simulink model "model_FS_PSH_IEEE39"  (R2020b)
settings: Solver=ode3  StartTime=0.0  StopTime=300  FixedStep=Ts  RelTol=1e-3
PostLoadFcn:
  | IEEE39BusLineLength;
  | vNomHV = 345E3;fNom=60;load('Dynamicload.mat');
InitFcn:
  | IEEE39BusLineLength;
  | vNomHV = 345E3;fNom=60;load('Dynamicload.mat');
values from neighbouring files (symbols this model uses):
  Rp = 0.05    [IEEE39BusLineLength.m]
  t_sw_off = 220    [MAIN_FS_PSH_IEEE39.m]    (also in MAIN_T_PSH_IEEE39.m; MAIN_VS_PSH.m = 45)
  t_sw_on = 130    [MAIN_FS_PSH_IEEE39.m]    (also in MAIN_T_PSH_IEEE39.m; MAIN_VS_PSH.m = 35)
  TL_10_11_len = 14    [IEEE39BusLineLength.m]
  TL_10_13_len = 14    [IEEE39BusLineLength.m]
  TL_13_14_len = 32    [IEEE39BusLineLength.m]
  TL_14_15_len = 70    [IEEE39BusLineLength.m]
  TL_15_16_len = 31.5    [IEEE39BusLineLength.m]
  TL_16_17_len = 26    [IEEE39BusLineLength.m]
  TL_16_19_len = 61    [IEEE39BusLineLength.m]
  TL_16_21_len = 46    [IEEE39BusLineLength.m]
  TL_16_24_len = 15    [IEEE39BusLineLength.m]
  TL_17_18_len = 26    [IEEE39BusLineLength.m]
  TL_17_27_len = 59    [IEEE39BusLineLength.m]
  TL_1_2_len = 134    [IEEE39BusLineLength.m]
  TL_1_39_len = 105    [IEEE39BusLineLength.m]
  TL_21_22_len = 47    [IEEE39BusLineLength.m]
  TL_22_23_len = 33    [IEEE39BusLineLength.m]
  TL_24_23_len = 88    [IEEE39BusLineLength.m]
  TL_25_26_len = 101    [IEEE39BusLineLength.m]
  TL_26_27_len = 46.5    [IEEE39BusLineLength.m]
  TL_26_28_len = 151    [IEEE39BusLineLength.m]
  TL_26_29_len = 200    [IEEE39BusLineLength.m]
  TL_28_29_len = 48    [IEEE39BusLineLength.m]
  TL_2_25_len = 28    [IEEE39BusLineLength.m]
  TL_2_2_len = 49    [IEEE39BusLineLength.m]
  TL_3_18_len = 42    [IEEE39BusLineLength.m]
  TL_3_4_len = 53    [IEEE39BusLineLength.m]
  TL_4_14_len = 33    [IEEE39BusLineLength.m]
  TL_4_5_len = 32.5    [IEEE39BusLineLength.m]
  TL_5_6_len = 14    [IEEE39BusLineLength.m]
  TL_5_8_len = 32    [IEEE39BusLineLength.m]
  TL_6_11_len = 26.5    [IEEE39BusLineLength.m]
  TL_6_7_len = 25.5    [IEEE39BusLineLength.m]
  TL_7_8_len = 15    [IEEE39BusLineLength.m]
  TL_8_9_len = 93    [IEEE39BusLineLength.m]
  TL_9_39_len = 136    [IEEE39BusLineLength.m]
  Ts = 25e-6    (= 2.5e-05)    [MAIN_FS_PSH_IEEE39.m]    (also in MAIN_T_PSH_IEEE39.m; MAIN_VS_PSH.m = 1e-07)
undefined symbols (not defined in the file or in its folder): D1, Delta, FS_PSH, load15, load16, load18, load20, load21, load23, load24, load25, load26, load27, load28, load29, load3, load39, load4, load7, load8
libraries: powerlib x216, sps_avr x10, powerlib_meascontrol x5, pid_lib x1
(part 4 of 8)

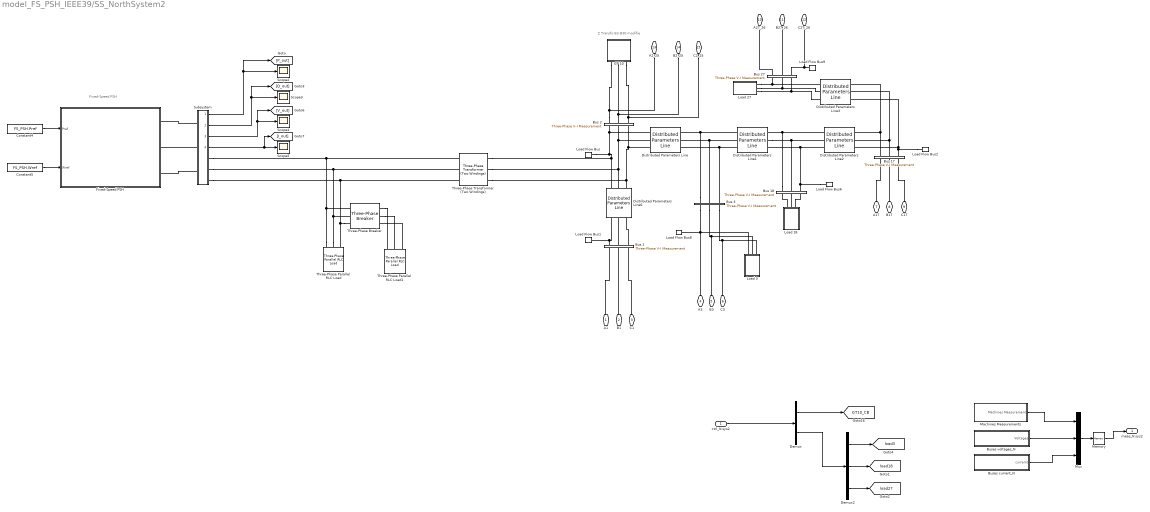
== system model_FS_PSH_IEEE39/SS_NorthSystem2 ==
  note: Z Transfo B2-B30 modifie
  note: Fixed-Speed PSH
  ctrl_N sys2 : Inport
  Bus 1 : powerlib/Measurements/Three-Phase V-I Measurement  VoltageMeasurement=phase-to-ground  SetLabelV=on  LabelV=V_bus_1  Vpu=off  VpuLL=off  CurrentMeasurement=yes  SetLabelI=on  LabelI=I_bus_1  Ipu=off  Pbase=100e6  Vbase=230e3  OutputType=Complex  PhasorSimulation=off  PSBequivalent=0
  Bus 17 : powerlib/Measurements/Three-Phase V-I Measurement  VoltageMeasurement=phase-to-ground  SetLabelV=on  LabelV=V_bus_17  Vpu=off  VpuLL=off  CurrentMeasurement=yes  SetLabelI=on  LabelI=I_bus_17  Ipu=off  Pbase=100e6  Vbase=230e3  OutputType=Complex  PhasorSimulation=off  PSBequivalent=0
  Bus 18 : powerlib/Measurements/Three-Phase V-I Measurement  VoltageMeasurement=phase-to-ground  SetLabelV=on  LabelV=V_bus_18  Vpu=off  VpuLL=off  CurrentMeasurement=yes  SetLabelI=on  LabelI=I_bus_18  Ipu=off  Pbase=100e6  Vbase=230e3  OutputType=Complex  PhasorSimulation=off  PSBequivalent=0
  Bus 2 : powerlib/Measurements/Three-Phase V-I Measurement  VoltageMeasurement=phase-to-ground  SetLabelV=on  LabelV=V_bus_2  Vpu=off  VpuLL=off  CurrentMeasurement=yes  SetLabelI=on  LabelI=I_bus_2  Ipu=off  Pbase=100e6  Vbase=230e3  OutputType=Complex  PhasorSimulation=off  PSBequivalent=0
  Bus 27 : powerlib/Measurements/Three-Phase V-I Measurement  VoltageMeasurement=phase-to-ground  SetLabelV=on  LabelV=V_bus_27  Vpu=off  VpuLL=off  CurrentMeasurement=yes  SetLabelI=on  LabelI=I_bus_27  Ipu=off  Pbase=100e6  Vbase=230e3  OutputType=Complex  PhasorSimulation=off  PSBequivalent=0
  Bus 3 : powerlib/Measurements/Three-Phase V-I Measurement  VoltageMeasurement=phase-to-ground  SetLabelV=on  LabelV=V_bus_3  Vpu=off  VpuLL=off  CurrentMeasurement=yes  SetLabelI=on  LabelI=I_bus_3  Ipu=off  Pbase=100e6  Vbase=230e3  OutputType=Complex  PhasorSimulation=off  PSBequivalent=0
  Buses current_N : Subsystem
  Buses voltages_N : Subsystem
  Constant4 : Constant  Value=FS_PSH.Pref
  Constant5 : Constant  Value=FS_PSH.Wref
  Demux : Demux  Outputs=[1 6]
  Demux2 : Demux  Outputs=[2 2 2]
  Distributed Parameters Line : powerlib/Elements/Distributed Parameters Line  Phases=3  Length=TL_2_2_len  Frequency=fNom  Resistance=[1.547 6.189]/TL_2_2_len  Inductance="[0.048  0.143]/TL_2_2_len"  Capacitance=[0.573e-6 0.261e-6]/TL_2_2_len  x1=[-0.0002 -1.51494241435871e-08 0 0;-0.000175 -1.51813366174431e-08 204759.764947038 -188224.30962879;-0.00015 -1.52119005972007e-08 206524.605301447 -186286.162393846;-0.000125 -1.52411133679905e-08 208271.100946267 -184331.468144834;-0.0001 -1.52689723349653e-08 209999.096747657 -182360.400508997;-7.5e-05 -1.52954750235306e-08 211708.439215037 -180373.134567961;-5e-05 -1.53206190795644e-08 213398.976514727 -178369.846842178;-2.5e-05 -1.53444022696261e-08 215070.558483429 -176350.715275245]  x2=[-0.0002 7.17563772164822e-10 0 0;-0.000175 6.09800920547567e-10 182393.138299879 -200537.913661572;-0.00015 5.0198390288662e-10 184275.023772651 -198810.016888842;-0.000125 3.94122296112896e-10 186140.540872315 -197064.460660873;-0.0001 2.86225681117977e-10 187989.523892855 -195301.400028062;-7.5e-05 1.78303641903076e-10 189821.808596909 -193520.991595647;-5e-05 7.03657647277308e-11 191637.232230355 -191723.393509802;-2.5e-05 -3.75783627416992e-11 193435.633536768 -189908.765443581]  x3=[-0.0002 1.59600858713236e-10 0 0;-0.000175 1.6212940524219e-10 -94.4406795368501 497.211528971884;-0.00015 1.64643550499921e-10 -99.1225635679205 496.299405662674;-0.000125 1.67143071165511e-10 -103.795642959758 495.3431981706;-0.0001 1.69627745217082e-10 -108.459502622431 494.342991431541;-7.5e-05 1.72097351951519e-10 -113.113728284958 493.298874289642;-5e-05 1.74551672004071e-10 -117.757906532103 492.210939489424;-2.5e-05 1.7699048736784e-10 -122.391624841103 491.079283667549]  x4=[-0.0002 -1.7528128884237e-10 0 0;-0.000175 -1.77995252123788e-10 1384.83776478724 -1876.75500949724;-0.00015 -1.80693404837725e-10 1402.46395776973 -1863.6200869169;-0.000125 -1.83375507318658e-10 1419.9655757943 -1850.31962682479;-0.0001 -1.86041321326734e-10 1437.34106426604 -1836.8548106447;-7.5e-05 -1.88690610068941e-10 1454.5888797936 -1823.22683439944;-5e-05 -1.91323138220134e-10 1471.70749032629 -1809.43690860468;-2.5e-05 -1.9393867194394e-10 1488.69537529012 -1795.48625816134]  x5=0.000193191614724863  V1=ones(3,3)  V2=ones(3,3)  I1=ones(3,3)  I2=ones(3,3)  nHarmo=1  Measurements=None  Decoupling=off  VsMag0=0  VrMag0=0  VsAngle0=0  VrAngle0=0  IsMag0=0  IrMag0=0  IsAngle0=0  IrAngle0=0
  Distributed Parameters Line1 : powerlib/Elements/Distributed Parameters Line  Phases=3  Length=TL_3_18_len  Frequency=fNom  Resistance=[1.309 5.237]/TL_3_18_len  Inductance=[0.042 0.126]/TL_3_18_len  Capacitance=[0.476e-6 0.217e-6]/TL_3_18_len  x1=[-0.000175 6.10040756475759e-10 182393.138299879 -200537.913661572;-0.00015 5.02189516117273e-10 184275.023772651 -198810.016888842;-0.000125 3.94293668382255e-10 186140.540872315 -197064.460660873;-0.0001 2.86362797203766e-10 187989.523892855 -195301.400028062;-7.5e-05 1.7840648962585e-10 189821.808596909 -193520.991595647;-5e-05 7.04343349519622e-11 191637.232230355 -191723.393509802;-2.5e-05 -3.75440761068149e-11 193435.633536768 -189908.765443581]  x2=[-0.000175 1.38990555358626e-08 174480.81486006 -206839.81724275;-0.00015 1.36965263186684e-08 176422.445257544 -205186.21137713;-0.000125 1.34927804968119e-08 178348.404793348 -203514.379685809;-0.0001 1.3287836168175e-08 180258.52239261 -201824.470670543;-7.5e-05 1.30817115370981e-08 182152.62838764 -200116.634438822;-5e-05 1.28744249127627e-08 184030.554532992 -198391.022690537;-2.5e-05 1.26659947075654e-08 185892.134020407 -196647.788704499]  x3=[-0.000175 2.40901588856487e-10 158.479314501855 -226.352731913089;-0.00015 2.43141653382429e-10 160.605532962627 -224.84904453694;-0.000125 2.45360120660848e-10 162.717485511325 -223.325384768556;-0.0001 2.47556793634653e-10 164.81498455211 -221.781887948207;-7.5e-05 2.4973147718265e-10 166.897843772991 -220.218691178206;-5e-05 2.5188397813687e-10 168.965878162367 -218.635933310727;-2.5e-05 2.54014105299734e-10 171.018904025468 -217.033754935477]  x4=[-0.000175 -2.1821723930702e-10 1002.49352677277 -1172.51684770348;-0.00015 -2.20849624055767e-10 1013.4995116839 -1163.01665378402;-0.000125 -2.23462391663931e-10 1024.41547170825 -1153.41315400069;-0.0001 -2.26055310050386e-10 1035.24043722713 -1143.70720139188;-7.5e-05 -2.28628148897127e-10 1045.9734467045 -1133.89965809641;-5e-05 -2.31180679669733e-10 1056.61354677242 -1123.99139527698;-2.5e-05 -2.3371267563766e-10 1067.15979231567 -1113.9832930428]  x5=0.000165354165354248  V1=ones(3,3)  V2=ones(3,3)  I1=ones(3,3)  I2=ones(3,3)  nHarmo=1  Measurements=None  Decoupling=off  VsMag0=0  VrMag0=0  VsAngle0=0  VrAngle0=0  IsMag0=0  IrMag0=0  IsAngle0=0  IrAngle0=0
  Distributed Parameters Line2 : powerlib/Elements/Distributed Parameters Line  Phases=3  Length=TL_17_18_len  Frequency=fNom  Resistance=[0.833 3.333]/TL_17_18_len  Inductance=[0.026 0.078]/TL_17_18_len  Capacitance=[0.294e-6 0.134e-6]/TL_17_18_len  x1=[-0.000125 1.34927804968119e-08 0 0;-0.0001 1.3287836168175e-08 180258.52239261 -201824.470670543;-7.5e-05 1.30817115370981e-08 182152.62838764 -200116.634438822;-5e-05 1.28744249127627e-08 184030.554532992 -198391.022690537;-2.5e-05 1.26659947075654e-08 185892.134020407 -196647.788704499]  x2=[-0.000125 2.16125954865691e-08 0 0;-0.0001 2.13654534678538e-08 179085.783169739 -203138.687259504;-7.5e-05 2.11164136460244e-08 180992.327499674 -201441.845312146;-5e-05 2.08654981422377e-08 182882.795044564 -199727.110135331;-2.5e-05 2.06127292442597e-08 184757.017882151 -197994.634041752]  x3=[-0.000125 1.96642687638485e-10 0 0;-0.0001 1.98777681586451e-10 450.672583897956 -579.878942450258;-7.5e-05 2.00895018951385e-10 456.117684022584 -575.605735092421;-5e-05 2.02994511659141e-10 461.5222691372 -571.281399104982;-2.5e-05 2.05075973220637e-10 466.885859175303 -566.906318600468]  x4=[-0.000125 -1.52053953043735e-10 0 0;-0.0001 -1.54749878520997e-10 732.742892591496 -798.917316240247;-7.5e-05 -1.5743205821927e-10 740.239817501564 -791.97601728488;-5e-05 -1.60100253891843e-10 747.670990030899 -784.964370440372;-2.5e-05 -1.62754228534151e-10 755.035750099792 -777.882998521739]  x5=0.000102235023353056  V1=ones(3,3)  V2=ones(3,3)  I1=ones(3,3)  I2=ones(3,3)  nHarmo=1  Measurements=None  Decoupling=off  VsMag0=0  VrMag0=0  VsAngle0=0  VrAngle0=0  IsMag0=0  IrMag0=0  IsAngle0=0  IrAngle0=0
  Distributed Parameters Line3 : powerlib/Elements/Distributed Parameters Line  Phases=3  Length=TL_17_27_len  Frequency=fNom  Resistance=[1.547 6.189]/TL_17_27_len  Inductance=[0.055 0.164]/TL_17_27_len  Capacitance=[0.717e-6 0.326e-6]/TL_17_27_len  x1=[-0.00025 1.26915307639565e-08 0 0;-0.000225 1.2415117490423e-08 0 0;-0.0002 1.21376014343686e-08 173522.997948791 -209344.124994062;-0.000175 1.18590072463739e-08 175488.272737464 -207699.435035008;-0.00015 1.15793596727857e-08 177437.959643062 -206036.296011196;-0.000125 1.12986835535183e-08 179371.88548312 -204354.855652249;-0.0001 1.10170038198476e-08 181289.878475163 -202655.263313423;-7.5e-05 1.07343454921961e-08 183191.768251964 -200937.669962337;-5e-05 1.0450733677911e-08 185077.385876676 -199202.228165563;-2.5e-05 1.01661935690334e-08 186946.563857838 -197449.092075075]  x2=[-0.00025 2.281907620188e-08 0 0;-0.000225 2.25817490480763e-08 0 0;-0.0002 2.23424160527522e-08 171302.246109104 -209744.132408951;-0.000175 2.21010984748482e-08 173271.390022366 -208120.354518787;-0.00015 2.18578177495869e-08 175225.142968893 -206478.090175362;-0.000125 2.16125954865691e-08 177163.331405052 -204817.485254091;-0.0001 2.13654534678538e-08 179085.783169739 -203138.687259504;-7.5e-05 2.11164136460244e-08 180992.327499674 -201441.845312146;-5e-05 2.08654981422377e-08 182882.795044564 -199727.110135331;-2.5e-05 2.06127292442597e-08 184757.017882151 -197994.634041752]  x3=[-0.00025 -3.28342109599023e-11 0 0;-0.000225 -3.16222228881237e-11 0 0;-0.0002 -3.04074259476653e-11 568.598236759176 -671.205359816578;-0.000175 -2.91899280438154e-11 574.898815454013 -665.816688181209;-0.00015 -2.79698373217776e-11 581.148328311938 -660.368874857778;-0.000125 -2.67472621570644e-11 587.346220215085 -654.862403752562;-0.0001 -2.55223111458711e-11 593.491940630857 -649.297763982165;-7.5e-05 -2.42950930954292e-11 599.584943660833 -643.675449830066;-5e-05 -2.3065717014342e-11 605.624688089252 -637.995960702717;-2.5e-05 -2.18342921029012e-11 611.610637431093 -632.259801085182]  x4=[-0.00025 8.40639866488944e-11 0 0;-0.000225 8.21629601094671e-11 0 0;-0.0002 8.02546353808483e-11 614.710110599397 -882.118942511795;-0.000175 7.83391819714747e-11 622.996418676087 -876.286370108353;-0.00015 7.64167700229933e-11 631.227388608642 -870.375960882743;-0.000125 7.44875702951491e-11 639.40228927472 -864.388239831685;-0.0001 7.25517541506166e-11 647.520394532377 -858.323738819187;-7.5e-05 7.06094935397789e-11 655.580983284563 -852.182996529292;-5e-05 6.86609609854539e-11 663.583339543179 -845.966558418238;-2.5e-05 6.67063295675696e-11 671.526752492672 -839.674976666001]  x5=0.000231222836242444  V1=ones(3,3)  V2=ones(3,3)  I1=ones(3,3)  I2=ones(3,3)  nHarmo=1  Measurements=None  Decoupling=off  VsMag0=0  VrMag0=0  VsAngle0=0  VrAngle0=0  IsMag0=0  IrMag0=0  IsAngle0=0  IrAngle0=0
  Distributed Parameters Line6 : powerlib/Elements/Distributed Parameters Line  Phases=3  Length=TL_1_2_len  Frequency=fNom  Resistance=[4.166 16.66]/TL_1_2_len  Inductance=[0.13 0.389]/TL_1_2_len  Capacitance=[1.56e-6 0.708e-6]/TL_1_2_len  x1=[-0.000525 -1.4613301103022e-08 274028.296588638 -47576.3438444088;-0.0005 -1.46624428221208e-08 273567.731050763 -50156.8379538991;-0.000475 -1.47102821382683e-08 273082.86564522 -52732.8768430305;-0.00045 -1.47568148021e-08 272573.743440558 -55304.2316931339;-0.000425 -1.48020366803156e-08 272040.409659955 -57870.6741016037;-0.0004 -1.48459437560464e-08 271482.911677201 -60431.9761021857;-0.000375 -1.48885321292121e-08 270901.299012491 -62987.9101852266;-0.00035 -1.4929798016867e-08 270295.623328023 -65538.2493178824;-0.000325 -1.49697377535365e-08 269665.938423416 -68082.7669642851;-0.0003 -1.50083477915422e-08 269012.300230921 -70621.2371056646;-0.000275 -1.50456247013173e-08 268334.766810465 -73153.4342604253;-0.00025 -1.50815651717111e-08 267633.398344481 -75679.1335041745;-0.000225 -1.51161660102832e-08 266908.257132574 -78198.1104897015;-0.0002 -1.51494241435871e-08 266159.407585977 -80710.1414669055;-0.000175 -1.51813366174431e-08 265386.916221839 -83215.0033026703;-0.00015 -1.52119005972007e-08 264590.851657308 -85712.4735006842;-0.000125 -1.52411133679905e-08 263771.284603441 -88202.3302212036;-0.0001 -1.52689723349653e-08 262928.287858924 -90684.3523007581;-7.5e-05 -1.52954750235306e-08 262061.936303602 -93158.3192717952;-5e-05 -1.53206190795644e-08 261172.306891829 -95624.0113822638;-2.5e-05 -1.53444022696261e-08 260259.478645633 -98081.2096151338]  x2=[-0.000525 -1.83506064239342e-09 277953.853015804 -36021.720162291;-0.0005 -1.83453097485514e-09 277602.010942514 -38639.7239747498;-0.000475 -1.83383835366822e-09 277225.510653489 -41254.2955835064;-0.00045 -1.8329828403553e-09 276824.385591662 -43865.2027471928;-0.000425 -1.83196451090801e-09 276398.671387281 -46472.2135499382;-0.0004 -1.83078345578025e-09 275948.405854742 -49075.0964219691;-0.000375 -1.82943977988018e-09 275473.628989234 -51673.6201601786;-0.00035 -1.82793360256085e-09 274974.382963182 -54267.5539486635;-0.000325 -1.82626505760965e-09 274450.712122507 -56856.6673792262;-0.0003 -1.82443429323639e-09 273902.662982679 -59440.7304718413;-0.000275 -1.82244147206013e-09 273330.284224592 -62019.5136950836;-0.00025 -1.82028677109479e-09 272733.626690238 -64592.7879865165;-0.000225 -1.81797038173336e-09 272112.743378187 -67160.3247730384;-0.0002 -1.81549250973094e-09 271467.689438887 -69721.8959911863;-0.000175 -1.81285337518644e-09 270798.522169757 -72277.2741073932;-0.00015 -1.81005321252306e-09 270105.301010104 -74826.2321381994;-0.000125 -1.80709227046743e-09 269388.087535839 -77368.5436704144;-0.0001 -1.80397081202756e-09 268646.94545401 -79903.9828812278;-7.5e-05 -1.80068911446941e-09 267881.940597142 -82432.3245582689;-5e-05 -1.79724746929236e-09 267093.14091739 -84953.3441196108;-2.5e-05 -1.79364618220321e-09 266280.616480503 -87466.8176337191]  x3=[-0.000525 -4.48229179644309e-11 726.128281654629 16.226456823734;-0.0005 -4.4066576103207e-11 726.2489534958 9.3822847971849;-0.000475 -4.33063199938962e-11 726.305115705676 2.53727938185078;-0.00045 -4.25422171668421e-11 726.296763295607 -4.30795140930883;-0.000425 -4.17743354940758e-11 726.223897007501 -11.1527995433153;-0.0004 -4.10027431832876e-11 726.086523313763 -17.9966570211796;-0.000375 -4.02275087717678e-11 725.884654416719 -24.838915931909;-0.00035 -3.94487011203195e-11 725.618308247532 -31.6789685065041;-0.000325 -3.86663894071413e-11 725.287508464608 -38.5162071719455;-0.0003 -3.7880643121683e-11 724.892284451498 -45.3500246051613;-0.000275 -3.70915320584729e-11 724.432671314283 -52.1798137869733;-0.00025 -3.62991263109185e-11 723.908709878459 -59.0049680560158;-0.000225 -3.55034962650799e-11 723.32044668531 -65.8248811626229;-0.0002 -3.47047125934183e-11 722.667933987776 -72.6389473226791;-0.000175 -3.3902846248518e-11 721.951229745806 -79.4465612714284;-0.00015 -3.30979684567842e-11 721.170397621216 -86.2471183172375;-0.000125 -3.22901507121164e-11 720.32550697203 -93.0400143953083;-0.0001 -3.14794647695574e-11 719.41663284632 -99.8246461213337;-7.5e-05 -3.06659826389201e-11 718.443855975541 -106.600410845095;-5e-05 -2.9849776578391e-11 717.40726276736 -113.36670670399;-2.5e-05 -2.90309190881119e-11 716.306945297979 -120.122932676498]  x4=[-0.000525 2.39683517601749e-11 1189.83684018121 -141.162916344656;-0.0005 2.31103056027443e-11 1188.45356254151 -152.370397416942;-0.000475 2.2250206654344e-11 1186.96471958462 -163.564344069507;-0.00045 2.13881313139357e-11 1185.37044355819 -174.743761991287;-0.000425 2.05241561560358e-11 1183.67087607504 -185.907658161741;-0.0004 1.96583579239134e-11 1181.86616810057 -197.05504093906;-0.000375 1.87908135227736e-11 1179.95647993937 -208.184920148251;-0.00035 1.79216000129263e-11 1177.94198122101 -219.296307169088;-0.000325 1.70507946029414e-11 1175.82285088489 -230.388215023929;-0.0003 1.61784746427904e-11 1173.59927716443 -241.459658465385;-0.000275 1.53047176169762e-11 1171.27145757031 -252.509654063831;-0.00025 1.44296011376497e-11 1168.83959887291 -263.537220294767;-0.000225 1.35532029377168e-11 1166.30391708399 -274.541377625998;-0.0002 1.2675600863933e-11 1163.66463743748 -285.521148604642;-0.000175 1.17968728699889e-11 1160.92199436943 -296.475557943955;-0.00015 1.09170970095857e-11 1158.07623149729 -307.40363260996;-0.000125 1.00363514295024e-11 1155.12760159814 -318.304401907878;-0.0001 9.15471436265399e-12 1152.07636658636 -329.176897568351;-7.5e-05 8.27226412114237e-12 1148.92279749028 -340.020153833448;-5e-05 7.38907908930044e-12 1145.66717442814 -350.833207542451;-2.5e-05 6.50523771672941e-12 1142.3097865832 -361.615098217406]  x5=0.000524797103650544  V1=ones(3,3)  V2=ones(3,3)  I1=ones(3,3)  I2=ones(3,3)  nHarmo=1  Measurements=None  Decoupling=off  VsMag0=0  VrMag0=0  VsAngle0=0  VrAngle0=0  IsMag0=0  IrMag0=0  IsAngle0=0  IrAngle0=0
  Fixed-Speed PSH : Subsystem
  GT 10 : Subsystem
  Load 18 : Subsystem  SystemSampleTime=20e-3
  Load 27 : Subsystem  SystemSampleTime=20e-3
  Load 3 : Subsystem  SystemSampleTime=20e-3
  Load Flow Bus : powerlib/Measurements/Load Flow Bus  LConnTagsString=a  Phases=single  Connectors=on one side  ID=Bus-2  Vbase=345e+003  Vref=1  Vangle=0  VLF=1.028  VLFb=1  VLFc=1  angleLF=24.05  angleLFb=0  angleLFc=0
      settings: AttributesFormatString=%<ID>\n%<Vbase>V\n%<VLF>pu\n%<angleLF>deg.
  Load Flow Bus1 : powerlib/Measurements/Load Flow Bus  LConnTagsString=a  Phases=single  Connectors=on one side  ID=Bus-1  Vbase=345e+003  Vref=1  Vangle=0  VLF=1.036  VLFb=1  VLFc=1  angleLF=22.64  angleLFb=0  angleLFc=0
      settings: AttributesFormatString=%<ID>\n%<Vbase>V\n%<VLF>pu\n%<angleLF>deg.
  Load Flow Bus2 : powerlib/Measurements/Load Flow Bus  LConnTagsString=a  Phases=single  Connectors=on one side  ID=Bus-17  Vbase=345e+003  Vref=1  Vangle=0  VLF=1.01  VLFb=1  VLFc=1  angleLF=19.53  angleLFb=0  angleLFc=0
      settings: AttributesFormatString=%<ID>\n%<Vbase>V\n%<VLF>pu\n%<angleLF>deg.
  Load Flow Bus6 : powerlib/Measurements/Load Flow Bus  LConnTagsString=a  Phases=single  Connectors=on one side  ID=Bus-18  Vbase=345e+003  Vref=1  Vangle=0  VLF=1.009  VLFb=1  VLFc=1  angleLF=19.72  angleLFb=0  angleLFc=0
      settings: AttributesFormatString=%<ID>\n%<Vbase>V\n%<VLF>pu\n%<angleLF>deg.
  Load Flow Bus8 : powerlib/Measurements/Load Flow Bus  LConnTagsString=a  Phases=single  Connectors=on one side  ID=Bus-3  Vbase=345e+003  Vref=1  Vangle=0  VLF=1.01  VLFb=1  VLFc=1  angleLF=21  angleLFb=0  angleLFc=0
      settings: AttributesFormatString=%<ID>\n%<Vbase>V\n%<VLF>pu\n%<angleLF>deg.
  Load Flow Bus9 : powerlib/Measurements/Load Flow Bus  LConnTagsString=a  Phases=single  Connectors=on one side  ID=Bus-27  Vbase=345e+003  Vref=1  Vangle=0  VLF=1.013  VLFb=1  VLFc=1  angleLF=19.76  angleLFb=0  angleLFc=0
      settings: AttributesFormatString=%<ID>\n%<Vbase>V\n%<VLF>pu\n%<angleLF>deg.
  Machines Measurements : Subsystem
      mask Display: disp('Machines Measurements')
  Memory : Memory
  Mux : Mux  Inputs=3
  Scope{2..5} (4 alike) : Scope
  Subsystem : Subsystem
  Three-Phase Parallel RLC Load : powerlib/Elements/Three-Phase Parallel RLC Load  LConnTagsString=A|B|C  Configuration=Y (grounded)  NominalVoltage=18e3  Vabc=[1e3 1e3 1e3]  Vabcp=[1e3 1e3 1e3]  NominalFrequency=60  UnbalancedPower=off  ActivePower=0.001e6  InductivePower=0  CapacitivePower=0  Pabc=[10e3 9e3 11e3]  QLabc=[100 90 110]  QCabc=[100 90 110]  Pabcp=[10e3 9e3 11e3]  QLabcp=[100 90 110]  QCabcp=[100 90 110]  Measurements=None  LoadType=constant Z
  Three-Phase Parallel RLC Load1 : powerlib/Elements/Three-Phase Parallel RLC Load  LConnTagsString=A|B|C  Configuration=Y (grounded)  NominalVoltage=18e3  Vabc=[1e3 1e3 1e3]  Vabcp=[1e3 1e3 1e3]  NominalFrequency=60  UnbalancedPower=off  ActivePower=300e6  InductivePower=0  CapacitivePower=0  Pabc=[10e3 9e3 11e3]  QLabc=[100 90 110]  QCabc=[100 90 110]  Pabcp=[10e3 9e3 11e3]  QLabcp=[100 90 110]  QCabcp=[100 90 110]  Measurements=None  LoadType=constant Z
  Three-Phase Transformer (Two Windings) : powerlib/Elements/Three-Phase Transformer (Two Windings)  Winding1Connection=Yg  Winding2Connection=Yg  CoreType=Three single-phase transformers  SetSaturation=off  Hysteresis=off  DataFile='hysteresis'  SetInitialFlux=off  Measurements=None  UNITS=pu  NominalPower=[1000e6 , 60 ]  Winding1=[18e3 , 0.002 , 0.08 ]  Winding2=[ 345e3 , 0.002 , 0.08 ]  Rm=500  Lm=500  L0=0.5  Saturation=[ 0,0 ; 0.0024,1.2 ; 1.0,1.52 ]  InitialFluxes=[ 0.8 , -0.8 , 0.7 ]  BreakLoop=off  DiscreteSolver=Trapezoidal iterative  DataType=off  TransfoNumber=1
  Three-Phase Breaker : powerlib/Elements/Three-Phase Breaker  InitialState=open  SwitchA=on  SwitchB=on  SwitchC=on  SwitchTimes=[t_sw_on t_sw_off]  External=off  BreakerResistance=0.01  SnubberResistance=1e6  SnubberCapacitance=inf  Measurements=None
  A1 : PMIOPort  Side=Left
  B1 : PMIOPort  Port=2  Side=Left
  C1 : PMIOPort  Port=3  Side=Left
  A3 : PMIOPort  Port=4  Side=Left
  B3 : PMIOPort  Port=5  Side=Left
  C3 : PMIOPort  Port=6  Side=Left
  A17 : PMIOPort  Port=7  Side=Left
  B17 : PMIOPort  Port=8  Side=Left
  C17 : PMIOPort  Port=9  Side=Left
  A27_26 : PMIOPort  Port=10  Side=Right
  B27_26 : PMIOPort  Port=11  Side=Right
  C27_26 : PMIOPort  Port=12  Side=Right
  A2_25 : PMIOPort  Port=13  Side=Right
  B2_25 : PMIOPort  Port=14  Side=Right
  C2_25 : PMIOPort  Port=15  Side=Right
  meas_N sys2 : Outport
  tag scope: GT10_CB=global, load18=global, load27=global, load3=global
  wires:
  Machines Measurements/1(Machines Measurements) -> Mux/1
  Mux/1 -> Memory/1
  Memory/1 -> meas_N sys2/1
  Buses voltages_N/1(Voltages) -> Mux/2
  Buses current_N/1(curremt) -> Mux/3
  Demux/2 -> Demux2/1
  Demux/1 -> [GT10_CB]
  Demux2/1 -> [load3]
  Demux2/3 -> [load27]
  Demux2/2 -> [load18]
  ctrl_N sys2/1 -> Demux/1
  Subsystem/1(Out1) -> [P_out], Scope2/1
  Subsystem/2(Out2) -> [Q_out], Scope3/1
  Subsystem/3(Out3) -> [V_out], Scope4/1
  Subsystem/4(Out4) -> [I_out], Scope5/1
  Constant5/1 -> Fixed-Speed PSH/2(Wref)
  Constant4/1 -> Fixed-Speed PSH/1(Pref)
  connections:
  Load 27/LConn3 -- Distributed Parameters Line3/LConn3 -- Bus 27/LConn3
  Load 27/LConn2 -- Distributed Parameters Line3/LConn2 -- Bus 27/LConn2
  Load 27/LConn1 -- Distributed Parameters Line3/LConn1 -- Bus 27/LConn1
  GT 10/RConn3 -- C2_25/RConn1 -- Bus 2/RConn3
  GT 10/RConn2 -- B2_25/RConn1 -- Bus 2/RConn2
  Bus 2/RConn1 -- GT 10/RConn1 -- A2_25/RConn1
  Load 18/LConn3 -- Bus 18/LConn3
  Load 18/LConn2 -- Bus 18/LConn2
  Load 18/LConn1 -- Bus 18/LConn1
  Load Flow Bus2/LConn1 -- Distributed Parameters Line2/RConn3 -- Distributed Parameters Line3/RConn3 -- Bus 17/RConn3
  Distributed Parameters Line2/RConn2 -- Distributed Parameters Line3/RConn2 -- Bus 17/RConn2
  Distributed Parameters Line2/RConn1 -- Distributed Parameters Line3/RConn1 -- Bus 17/RConn1
  Bus 1/RConn3 -- Distributed Parameters Line6/RConn1
  Bus 1/RConn2 -- Distributed Parameters Line6/RConn2
  Load Flow Bus1/LConn1 -- Distributed Parameters Line6/RConn3 -- Bus 1/RConn1
  Bus 2/LConn3 -- Distributed Parameters Line6/LConn1 -- Three-Phase Transformer (Two Windings)/RConn3 -- Distributed Parameters Line/LConn3
  Distributed Parameters Line6/LConn3 -- Three-Phase Transformer (Two Windings)/RConn1 -- Load Flow Bus/LConn1 -- Distributed Parameters Line/LConn1 -- Bus 2/LConn1
  Distributed Parameters Line/RConn2 -- Distributed Parameters Line1/LConn2 -- Bus 3/RConn2
  Bus 3/RConn1 -- Distributed Parameters Line1/LConn1 -- Distributed Parameters Line/RConn1
  Distributed Parameters Line/RConn3 -- Bus 3/RConn3 -- Distributed Parameters Line1/LConn3
  Bus 3/LConn3 -- C3/RConn1 -- Load 3/LConn3
  Bus 3/LConn2 -- B3/RConn1 -- Load 3/LConn2
  Load Flow Bus8/LConn1 -- Load 3/LConn1 -- Bus 3/LConn1 -- A3/RConn1
  Bus 2/LConn2 -- Distributed Parameters Line6/LConn2 -- Three-Phase Transformer (Two Windings)/RConn2 -- Distributed Parameters Line/LConn2
  B1/RConn1 -- Bus 1/LConn2
  A1/RConn1 -- Bus 1/LConn1
  C1/RConn1 -- Bus 1/LConn3
  Bus 18/RConn1 -- Distributed Parameters Line1/RConn1 -- Distributed Parameters Line2/LConn1
  Bus 18/RConn2 -- Distributed Parameters Line1/RConn2 -- Distributed Parameters Line2/LConn2
  Load Flow Bus6/LConn1 -- Distributed Parameters Line1/RConn3 -- Distributed Parameters Line2/LConn3 -- Bus 18/RConn3
  Bus 17/LConn2 -- B17/RConn1
  Bus 17/LConn3 -- C17/RConn1
  Bus 17/LConn1 -- A17/RConn1
  Bus 27/RConn2 -- B27_26/RConn1
  Load Flow Bus9/LConn1 -- Bus 27/RConn3 -- C27_26/RConn1
  Bus 27/RConn1 -- A27_26/RConn1
  Three-Phase Breaker/LConn3 -- Three-Phase Parallel RLC Load/LConn3 -- Three-Phase Transformer (Two Windings)/LConn3 -- Subsystem/RConn3
  Three-Phase Parallel RLC Load/LConn2 -- Three-Phase Transformer (Two Windings)/LConn2 -- Subsystem/RConn2 -- Three-Phase Breaker/LConn2
  Three-Phase Parallel RLC Load/LConn1 -- Three-Phase Breaker/LConn1 -- Three-Phase Transformer (Two Windings)/LConn1 -- Subsystem/RConn1
  Subsystem/LConn1 -- Fixed-Speed PSH/RConn1
  Three-Phase Breaker/RConn1 -- Three-Phase Parallel RLC Load1/LConn1
  Subsystem/LConn3 -- Fixed-Speed PSH/RConn3
  Three-Phase Parallel RLC Load1/LConn3 -- Three-Phase Breaker/RConn3
  Subsystem/LConn2 -- Fixed-Speed PSH/RConn2
  Three-Phase Breaker/RConn2 -- Three-Phase Parallel RLC Load1/LConn2

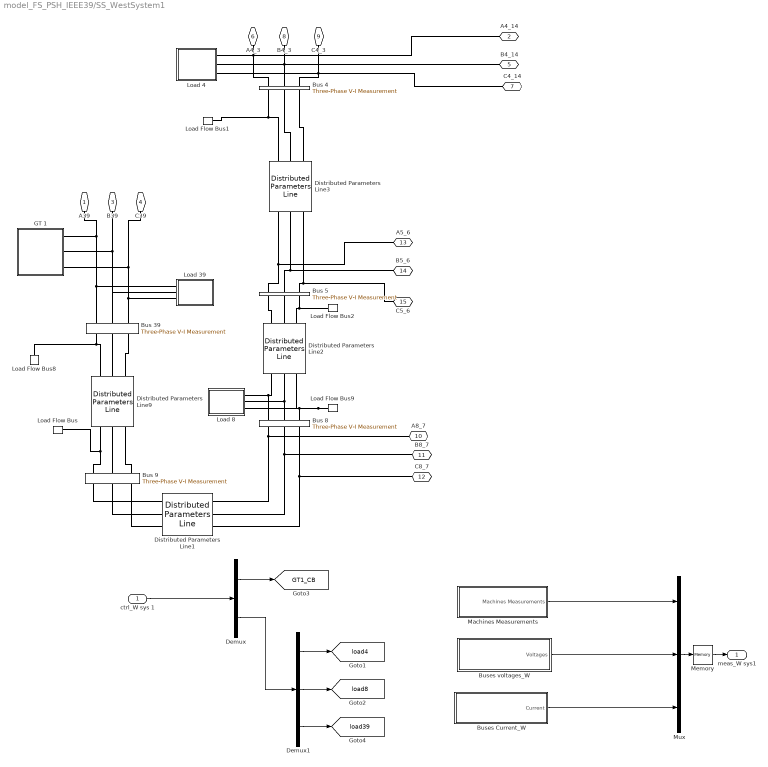
== system model_FS_PSH_IEEE39/SS_WestSystem1 ==
  ctrl_W sys 1 : Inport
  Bus 39 : powerlib/Measurements/Three-Phase V-I Measurement  VoltageMeasurement=phase-to-ground  SetLabelV=on  LabelV=V_bus_39  Vpu=off  VpuLL=off  CurrentMeasurement=yes  SetLabelI=on  LabelI=I_bus_39  Ipu=off  Pbase=100e6  Vbase=345e3  OutputType=Complex  PhasorSimulation=off  PSBequivalent=0
  Bus 4 : powerlib/Measurements/Three-Phase V-I Measurement  VoltageMeasurement=phase-to-ground  SetLabelV=on  LabelV=V_bus_4  Vpu=off  VpuLL=off  CurrentMeasurement=yes  SetLabelI=on  LabelI=I_bus_4  Ipu=off  Pbase=100e6  Vbase=230e3  OutputType=Complex  PhasorSimulation=off  PSBequivalent=0
  Bus 5 : powerlib/Measurements/Three-Phase V-I Measurement  VoltageMeasurement=phase-to-ground  SetLabelV=on  LabelV=V_bus_5  Vpu=off  VpuLL=off  CurrentMeasurement=yes  SetLabelI=on  LabelI=I_bus_5  Ipu=off  Pbase=100e6  Vbase=230e3  OutputType=Complex  PhasorSimulation=off  PSBequivalent=0
  Bus 8 : powerlib/Measurements/Three-Phase V-I Measurement  VoltageMeasurement=phase-to-ground  SetLabelV=on  LabelV=V_bus_8  Vpu=off  VpuLL=off  CurrentMeasurement=yes  SetLabelI=on  LabelI=I_bus_8  Ipu=off  Pbase=100e6  Vbase=230e3  OutputType=Complex  PhasorSimulation=off  PSBequivalent=0
  Bus 9 : powerlib/Measurements/Three-Phase V-I Measurement  VoltageMeasurement=phase-to-ground  SetLabelV=on  LabelV=V_bus_9  Vpu=off  VpuLL=off  CurrentMeasurement=yes  SetLabelI=on  LabelI=I_bus_9  Ipu=off  Pbase=100e6  Vbase=230e3  OutputType=Complex  PhasorSimulation=off  PSBequivalent=0
  Buses Current_W : Subsystem
  Buses voltages_W : Subsystem
  Demux : Demux  Outputs=[1 6]
  Demux1 : Demux  Outputs=[2 2 2]
  Distributed Parameters Line1 : powerlib/Elements/Distributed Parameters Line  Phases=3  Length=TL_8_9_len  Frequency=fNom  Resistance=[2.738 10.95]/TL_8_9_len  Inductance=[0.115 0.344]/TL_8_9_len  Capacitance=[0.848e-6 0.385e-6]/TL_8_9_len  x1=[-0.000375 7.55866534157526e-09 263003.047574398 -18768.6056536348;-0.00035 7.40722103418913e-09 262814.47331525 -21246.4710010015;-0.000325 7.25511877460145e-09 262602.554354963 -23722.4491139647;-0.0003 7.10237207341438e-09 262367.309517403 -26196.320061832;-0.000275 6.94899449847313e-09 262108.759698378 -28667.8641010816;-0.00025 6.79499967366073e-09 261826.927863778 -31136.8616948813;-0.000225 6.64040127768796e-09 261521.839047535 -33603.0935325888;-0.0002 6.48521304287823e-09 261193.520349402 -36066.3405492323;-0.000175 6.32944875394788e-09 260842.000932545 -38526.383944969;-0.00015 6.17312224678169e-09 260467.31202095 -40983.0052045202;-0.000125 6.01624740720394e-09 260069.486896653 -43435.9861165814;-0.0001 5.85883816974493e-09 259648.560896783 -45885.1087932044;-7.5e-05 5.70090851640329e-09 259204.571410419 -48330.1556891522;-5e-05 5.542472475404e-09 258737.557875276 -50770.9096212218;-2.5e-05 5.38354411995231e-09 258247.561774196 -53207.1537875364]  x2=[-0.000375 5.39280846269345e-09 272602.335386661 -34050.207643772;-0.00035 5.33621785614865e-09 272269.311055254 -36617.8634413172;-0.000325 5.27915325587932e-09 271912.10218935 -39182.2666285034;-0.0003 5.22161973069321e-09 271530.740518307 -41743.1894202118;-0.000275 5.16362239105069e-09 271125.259916873 -44300.4043404726;-0.00025 5.10516638861081e-09 270695.69640218 -46853.6842426705;-0.000225 5.04625691577371e-09 270242.088130542 -49402.8023297213;-0.0002 4.98689920521939e-09 269764.47539407 -51947.5321742171;-0.000175 4.92709852944291e-09 269262.900617088 -54487.6477385395;-0.00015 4.86686020028606e-09 268737.408352368 -57022.9233949366;-0.000125 4.80618956846556e-09 268188.045277172 -59553.1339455655;-0.0001 4.74509202309771e-09 267614.860189104 -62078.0546424952;-7.5e-05 4.68357299121977e-09 267017.904001778 -64597.46120767;-5e-05 4.62163793730786e-09 266397.229740294 -67111.1298528313;-2.5e-05 4.55929236279158e-09 265752.892536529 -69618.8372993958]  x3=[-0.000375 -6.87651886188109e-11 1077.6648573543 189.400069124221;-0.00035 -6.90071635517146e-11 1079.4020221404 179.235087698307;-0.000325 -6.92430088693453e-11 1081.04330819768 169.054185575549;-0.0003 -6.94727036225582e-11 1082.58856973763 158.85826708254;-0.000275 -6.96962274085372e-11 1084.03766950118 148.648237879714;-0.00025 -6.99135603726071e-11 1085.3904787709 138.425004880901;-0.000225 -7.01246832099976e-11 1086.64687738247 128.189476172767;-0.0002 -7.03295771675574e-11 1087.80675373528 117.942560934155;-0.000175 -7.05282240454205e-11 1088.87000480243 107.685169355324;-0.00015 -7.07206061986226e-11 1089.83653613978 97.4182125571057;-0.000125 -7.09067065386685e-11 1090.70626189446 87.1426025099658;-0.0001 -7.10865085350499e-11 1091.47910481238 76.8592519530036;-7.5e-05 -7.1259996216714e-11 1092.15499624517 66.5690743128751;-5e-05 -7.14271541734816e-11 1092.73387615624 56.272983622657;-2.5e-05 -7.15879675574165e-11 1093.21569312613 45.9718944406576]  x4=[-0.000375 8.40312166476196e-11 377.095665376244 -246.636976514389;-0.00035 8.4074561487233e-11 374.754422520639 -250.179988691063;-0.000325 8.41104383381675e-11 372.379891810358 -253.700778434576;-0.0003 8.41388440136337e-11 369.972284164948 -257.199033008025;-0.000275 8.41597759904755e-11 367.531813442041 -260.674441676212;-0.00025 8.41732324093935e-11 365.058696418359 -264.126695733243;-0.000225 8.41792120751108e-11 362.553152770455 -267.555488529952;-0.0002 8.4177714456479e-11 360.015405055203 -270.960515501137;-0.000175 8.41687396865251e-11 357.445678690029 -274.341474192615;-0.00015 8.41522885624402e-11 354.844201932887 -277.698064288084;-0.000125 8.41283625455082e-11 352.211205861985 -281.029987635806;-0.0001 8.40969637609762e-11 349.546924355257 -284.336948275082;-7.5e-05 8.40580949978659e-11 346.851594069593 -287.618652462547;-5e-05 8.40117597087256e-11 344.125454419812 -290.874808698261;-2.5e-05 8.39579620093235e-11 341.368747557402 -294.105127751599]  x5=0.000363923068793392  V1=ones(3,3)  V2=ones(3,3)  I1=ones(3,3)  I2=ones(3,3)  nHarmo=1  Measurements=None  Decoupling=off  VsMag0=0  VrMag0=0  VsAngle0=0  VrAngle0=0  IsMag0=0  IrMag0=0  IsAngle0=0  IrAngle0=0
  Distributed Parameters Line2 : powerlib/Elements/Distributed Parameters Line  Phases=3  Length=TL_5_8_len  Frequency=fNom  Resistance=[0.952 3.809]/TL_5_8_len  Inductance=[0.035 0.106]/TL_5_8_len  Capacitance=[0.329e-6 0.15e-6]/TL_5_8_len  x1=[-0.00015 6.17312224678169e-09 0 0;-0.000125 6.01624740720394e-09 167651.410863714 -203508.789343395;-0.0001 5.85883816974493e-09 169561.950318719 -201919.695396082;-7.5e-05 5.70090851640329e-09 171457.428300872 -200312.665773904;-5e-05 5.542472475404e-09 173337.67644286 -198687.843222525;-2.5e-05 5.38354411995231e-09 175202.52773017 -197045.372068077]  x2=[-0.00015 5.63994574386632e-09 0 0;-0.000125 5.48693110747864e-09 176044.303365788 -198561.861626215;-0.0001 5.33342909014401e-09 177907.847212146 -196893.887443867;-7.5e-05 5.17945332679916e-09 179755.588254834 -195208.424007976;-5e-05 5.02501749446172e-09 181587.362366807 -193505.62103115;-2.5e-05 4.87013531101526e-09 183403.006839299 -191785.629766195]  x3=[-0.00015 -4.0842485287564e-12 0 0;-0.000125 -4.38766064786698e-12 918.401437412413 -1238.13319400446;-0.0001 -4.69068302958892e-12 930.029574636806 -1229.42258821154;-7.5e-05 -4.99328875772218e-12 941.575101256855 -1220.60277799569;-5e-05 -5.29545095307628e-12 953.036991732129 -1211.67454678345;-2.5e-05 -5.5971427758579e-12 964.414227951241 -1202.63868763194]  x4=[-0.00015 1.60790522423646e-11 0 0;-0.000125 1.60201958674383e-11 108.144097102132 -13.182596356228;-0.0001 1.59599164860847e-11 108.263497307256 -12.1627988005452;-7.5e-05 1.58982194526669e-11 108.373280922557 -11.1419208747464;-5e-05 1.58351102474723e-11 108.473438196423 -10.1200532591118;-2.5e-05 1.57705944762253e-11 108.563960232303 -9.09728672183158]  x5=0.000126095202129185  V1=ones(3,3)  V2=ones(3,3)  I1=ones(3,3)  I2=ones(3,3)  nHarmo=1  Measurements=None  Decoupling=off  VsMag0=0  VrMag0=0  VsAngle0=0  VrAngle0=0  IsMag0=0  IrMag0=0  IsAngle0=0  IrAngle0=0
  Distributed Parameters Line3 : powerlib/Elements/Distributed Parameters Line  Phases=3  Length=TL_4_5_len  Frequency=fNom  Resistance=[0.952 3.809]/TL_4_5_len  Inductance=[0.04 0.121]/TL_4_5_len  Capacitance=[0.299e-6 0.136e-6]/TL_4_5_len  x1=[-0.00015 1.0331406401138e-09 0 0;-0.000125 8.56237621942703e-10 260371.90647512 -46555.6808839994;-0.0001 6.79258547795169e-10 259921.565620936 -49007.5153196876;-7.5e-05 5.02219137975879e-10 259448.1370304 -51454.9966244988;-5e-05 3.25135118148872e-10 258951.662756178 -53897.9073989918;-2.5e-05 1.48022217940708e-10 258432.186897986 -56336.0306497065]  x2=[-0.00015 5.63994574386632e-09 0 0;-0.000125 5.48693110747864e-09 259981.768073927 -53177.9080931996;-0.0001 5.33342909014401e-09 259469.031982336 -55625.7714963857;-7.5e-05 5.17945332679916e-09 258933.248351048 -58068.6938969137;-5e-05 5.02501749446172e-09 258374.464771464 -60506.4583002907;-2.5e-05 4.87013531101526e-09 257792.730877971 -62938.848170187]  x3=[-0.00015 -4.48054614826972e-11 0 0;-0.000125 -4.39941318341504e-11 1148.44196430186 -165.698808999273;-0.0001 -4.31788943724356e-11 1146.82928851537 -176.515044393957;-7.5e-05 -4.2359821511658e-11 1145.1147447204 -187.31560070177;-5e-05 -4.15369860066049e-11 1143.29848521263 -198.099518554851;-2.5e-05 -4.07104609462837e-11 1141.38067132274 -208.865840063263]  x4=[-0.00015 5.26649744080552e-11 0 0;-0.000125 5.15380607351429e-11 277.06818001458 -77.1523587723949;-0.0001 5.04065691536778e-11 276.328724445798 -79.7602056229134;-7.5e-05 4.92706001692847e-11 275.56472376195 -82.360967710787;-5e-05 4.8130254685297e-11 274.776245825994 -84.9544140212891;-2.5e-05 4.69856339937942e-11 273.9633606751 -87.5403141895229]  x5=0.000128280941686597  V1=ones(3,3)  V2=ones(3,3)  I1=ones(3,3)  I2=ones(3,3)  nHarmo=1  Measurements=None  Decoupling=off  VsMag0=0  VrMag0=0  VsAngle0=0  VrAngle0=0  IsMag0=0  IrMag0=0  IsAngle0=0  IrAngle0=0
  Distributed Parameters Line9 : powerlib/Elements/Distributed Parameters Line  Phases=3  Length=TL_9_39_len  Frequency=fNom  Resistance=[1.19 4.761]/TL_9_39_len  Inductance=[0.079 0.237]/TL_9_39_len  Capacitance=[2.674e-6 1.216e-6]/TL_9_39_len  x1=[-0.00055 5.77525405769042e-09 150987.568387585 -229508.672792301;-0.000525 5.72211974141417e-09 153143.886676562 -228075.476879521;-0.0005 5.66847715337662e-09 155286.601840032 -226622.021984128;-0.000475 5.61433105842261e-09 157415.523549643 -225148.437210392;-0.00045 5.55968626612136e-09 159530.46270226 -223654.853450632;-0.000425 5.50454763033928e-09 161631.231436759 -222141.403373593;-0.0004 5.44892004880884e-09 163717.643150714 -220608.221412663;-0.000375 5.39280846269345e-09 165789.512516972 -219055.443753928;-0.00035 5.33621785614865e-09 167846.655500117 -217483.208324079;-0.000325 5.27915325587932e-09 169888.889372814 -215891.654778156;-0.0003 5.22161973069321e-09 171916.032732043 -214280.924487149;-0.000275 5.16362239105069e-09 173927.905515208 -212651.160525435;-0.00025 5.10516638861081e-09 175924.329016137 -211002.507658072;-0.000225 5.04625691577371e-09 177905.125900951 -209335.112327942;-0.0002 4.98689920521939e-09 179870.120223817 -207649.122642738;-0.000175 4.92709852944291e-09 181819.137442577 -205944.688361813;-0.00015 4.86686020028606e-09 183752.004434253 -204221.960882875;-0.000125 4.80618956846556e-09 185668.549510423 -202481.09322854;-0.0001 4.74509202309771e-09 187568.602432471 -200722.240032737;-7.5e-05 4.68357299121977e-09 189451.994426711 -198945.557526979;-5e-05 4.62163793730786e-09 191318.558199375 -197151.203526479;-2.5e-05 4.55929236279158e-09 193168.127951477 -195339.337416133]  x2=[-0.00055 4.96715459497649e-09 160500.426952355 -225852.378290992;-0.000525 4.94959331633084e-09 162621.863287678 -224329.68964201;-0.0005 4.93159238618779e-09 164728.854608808 -222787.074732897;-0.000475 4.91315340349404e-09 166821.213760593 -221224.670587629;-0.00045 4.89427800610664e-09 168898.754887594 -219642.615987976;-0.000425 4.87496787064753e-09 170961.293450597 -218041.051461175;-0.0004 4.8552247123546e-09 173008.646243001 -216420.119267448;-0.000375 4.83505028492932e-09 175040.631407091 -214779.963387365;-0.00035 4.81444638038099e-09 177057.068450198 -213120.729509055;-0.000325 4.79341482886754e-09 179057.778260723 -211442.565015264;-0.0003 4.77195749853298e-09 181042.583124052 -209745.618970267;-0.000275 4.75007629534147e-09 183011.306738343 -208030.042106622;-0.00025 4.72777316290798e-09 184963.774230179 -206295.986811787;-0.000225 4.70505008232571e-09 186899.812170109 -204543.607114579;-0.0002 4.68190907199006e-09 188819.248588048 -202773.058671495;-0.000175 4.65835218741936e-09 190721.912988556 -200984.498752886;-0.00015 4.63438152107231e-09 192607.636365979 -199178.086228986;-0.000125 4.60999920216211e-09 194476.251219464 -197353.981555798;-0.0001 4.58520739646729e-09 196327.591567834 -195512.346760849;-7.5e-05 4.56000830613938e-09 198161.492964335 -193653.345428788;-5e-05 4.5344041695073e-09 199977.792511241 -191777.142686863;-2.5e-05 4.5083972608785e-09 201776.328874325 -189883.90519025]  x3=[-0.00055 -2.79038814988478e-11 893.748745600878 -1718.887617449;-0.000525 -2.80657788652775e-11 909.90887978608 -1710.38803386271;-0.0005 -2.82251832669492e-11 925.988190603395 -1701.73652372161;-0.000475 -2.83820805446422e-11 941.985249795463 -1692.93385550286;-0.00045 -2.85364567618333e-11 957.898636410992 -1683.98081111036;-0.000425 -2.86882982059341e-11 973.726936930968 -1674.87818580526;-0.0004 -2.88375913895096e-11 989.468745394219 -1665.62678813539;-0.000375 -2.89843230514761e-11 1005.1226635223 -1656.22743986337;-0.00035 -2.91284801582789e-11 1020.68730084368 -1646.68097589368;-0.000325 -2.92700499050502e-11 1036.16127481729 -1636.98824419842;-0.0003 -2.94090197167466e-11 1051.54321095528 -1627.15010574209;-0.000275 -2.95453772492658e-11 1066.83174294514 -1617.16743440502;-0.00025 -2.96791103905434e-11 1082.02551277106 -1607.04111690581;-0.000225 -2.98102072616286e-11 1097.12317083457 -1596.77205272251;-0.0002 -2.99386562177391e-11 1112.12337607436 -1586.3611540128;-0.000175 -3.00644458492961e-11 1127.02479608548 -1575.80934553289;-0.00015 -3.01875649829371e-11 1141.82610723764 -1565.11756455542;-0.000125 -3.03080026825088e-11 1156.5259947928 -1554.2867607862;-0.0001 -3.04257482500383e-11 1171.12315302196 -1543.31789627984;-7.5e-05 -3.05407912266835e-11 1185.61628532111 -1532.21194535432;-5e-05 -3.0653121393662e-11 1200.00410432645 -1520.96989450441;-2.5e-05 -3.07627287731589e-11 1214.2853320287 -1509.59274231407]  x4=[-0.00055 5.52237044534798e-11 679.75627178927 -1073.4634023423;-0.000525 5.52604990574033e-11 689.84301085178 -1067.00927225136;-0.0005 5.52923851042788e-11 699.868474069324 -1060.46036422731;-0.000475 5.53193597618032e-11 709.831770922292 -1053.81725998201;-0.00045 5.53414206339315e-11 719.732016413048 -1047.08054959441;-0.000425 5.53585657610895e-11 729.568331144544 -1040.25083145807;-0.0004 5.53707936203477e-11 739.339841398429 -1033.32871222804;-0.000375 5.53781031255571e-11 749.045679212665 -1026.31480676698;-0.00035 5.53804936274452e-11 758.684982458616 -1019.20973809054;-0.000325 5.53779649136737e-11 768.256894917632 -1012.01413731198;-0.0003 5.53705172088576e-11 777.760566357103 -1004.72864358617;-0.000275 5.53581511745451e-11 787.19515260598 -997.353904052805;-0.00025 5.53408679091589e-11 796.559815629762 -989.890573778878;-0.000225 5.53186689478986e-11 805.85372360493 -982.339315700542;-0.0002 5.52915562626042e-11 815.076050992841 -974.700800564201;-0.000175 5.52595322615812e-11 824.225978613051 -966.975706866936;-0.00015 5.52225997893866e-11 833.302693716083 -959.164720796236;-0.000125 5.51807621265761e-11 842.30539005562 -951.268536169048;-0.0001 5.51340229894128e-11 851.233267960118 -943.287854370148;-7.5e-05 5.50823865295371e-11 860.085534403839 -935.223384289837;-5e-05 5.5025857333598e-11 868.861403077293 -927.075842260978;-2.5e-05 5.49644404228455e-11 877.560094457083 -918.845951995365]  x5=0.000536835170233844  V1=ones(3,3)  V2=ones(3,3)  I1=ones(3,3)  I2=ones(3,3)  nHarmo=1  Measurements=None  Decoupling=off  VsMag0=0  VrMag0=0  VsAngle0=0  VrAngle0=0  IsMag0=0  IrMag0=0  IsAngle0=0  IrAngle0=0
  "GT 1 " : Subsystem
  Load 39 : Subsystem  SystemSampleTime=20e-3
  Load 4 : Subsystem
  Load 8 : Subsystem
  Load Flow Bus : powerlib/Measurements/Load Flow Bus  LConnTagsString=a  Phases=single  Connectors=on one side  ID=Bus-9  Vbase=345e+003  Vref=1  Vangle=0  VLF=1.022  VLFb=1  VLFc=1  angleLF=20.59  angleLFb=0  angleLFc=0
      settings: AttributesFormatString=%<ID>\n%<Vbase>V\n%<VLF>pu\n%<angleLF>deg.
  Load Flow Bus1 : powerlib/Measurements/Load Flow Bus  LConnTagsString=a  Phases=single  Connectors=on one side  ID=Bus-4  Vbase=345e+003  Vref=1  Vangle=0  VLF=0.9935  VLFb=1  VLFc=1  angleLF=19.16  angleLFb=0  angleLFc=0
      settings: AttributesFormatString=%<ID>\n%<Vbase>V\n%<VLF>pu\n%<angleLF>deg.
  Load Flow Bus2 : powerlib/Measurements/Load Flow Bus  LConnTagsString=a  Phases=single  Connectors=on one side  ID=Bus-5  Vbase=345e+003  Vref=1  Vangle=0  VLF=0.9982  VLFb=1  VLFc=1  angleLF=20.09  angleLFb=0  angleLFc=0
      settings: AttributesFormatString=%<ID>\n%<Vbase>V\n%<VLF>pu\n%<angleLF>deg.
  Load Flow Bus8 : powerlib/Measurements/Load Flow Bus  LConnTagsString=a  Phases=single  Connectors=on one side  ID=Bus-39  Vbase=345000  Vref=1.03  Vangle=0  VLF=1.029  VLFb=1  VLFc=1  angleLF=21.84  angleLFb=0  angleLFc=0
      settings: AttributesFormatString=%<ID>\n%<Vbase>V\n%<VLF>pu\n%<angleLF>deg.
  Load Flow Bus9 : powerlib/Measurements/Load Flow Bus  LConnTagsString=a  Phases=single  Connectors=on one side  ID=Bus-8  Vbase=345e+003  Vref=1  Vangle=0  VLF=0.9916  VLFb=1  VLFc=1  angleLF=18.81  angleLFb=0  angleLFc=0
      settings: AttributesFormatString=%<ID>\n%<Vbase>V\n%<VLF>pu\n%<angleLF>deg.
  Machines Measurements : Subsystem
      mask Display: disp('Machines Measurements')
  Memory : Memory
  Mux : Mux  Inputs=3
  A39 : PMIOPort  Side=Right
  A4_14 : PMIOPort  Port=2  Side=Left
  B39 : PMIOPort  Port=3  Side=Right
  C39 : PMIOPort  Port=4  Side=Right
  B4_14 : PMIOPort  Port=5  Side=Left
  A4_3 : PMIOPort  Port=6  Side=Right
  C4_14 : PMIOPort  Port=7  Side=Left
  B4_3 : PMIOPort  Port=8  Side=Right
  C4_3 : PMIOPort  Port=9  Side=Right
  A8_7 : PMIOPort  Port=10  Side=Left
  B8_7 : PMIOPort  Port=11  Side=Left
  C8_7 : PMIOPort  Port=12  Side=Left
  A5_6 : PMIOPort  Port=13  Side=Right
  B5_6 : PMIOPort  Port=14  Side=Right
  C5_6 : PMIOPort  Port=15  Side=Right
  meas_W sys1 : Outport
  tag scope: GT1_CB=global, load39=global, load4=global, load8=global
  wires:
  ctrl_W sys 1/1 -> Demux/1
  Mux/1 -> Memory/1
  Memory/1 -> meas_W sys1/1
  Buses voltages_W/1(Voltages) -> Mux/2
  Machines Measurements/1(Machines Measurements) -> Mux/1
  Buses Current_W/1(Current) -> Mux/3
  Demux/1 -> [GT1_CB]
  Demux/2 -> Demux1/1
  Demux1/2 -> [load8]
  Demux1/1 -> [load4]
  Demux1/3 -> [load39]
  connections:
  Distributed Parameters Line9/LConn3 -- Bus 9/RConn3
  Distributed Parameters Line9/LConn2 -- Bus 9/RConn2
  Bus 9/RConn1 -- Distributed Parameters Line9/LConn1 -- Load Flow Bus/LConn1
  Load Flow Bus9/LConn1 -- Distributed Parameters Line2/LConn3 -- Load 8/LConn3 -- Bus 8/RConn3
  Load 8/LConn2 -- Distributed Parameters Line2/LConn2 -- Bus 8/RConn2
  Load 8/LConn1 -- Distributed Parameters Line2/LConn1 -- Bus 8/RConn1
  Bus 8/LConn3 -- Distributed Parameters Line1/LConn1 -- C8_7/RConn1
  Bus 8/LConn2 -- Distributed Parameters Line1/LConn2 -- B8_7/RConn1
  A8_7/RConn1 -- Distributed Parameters Line1/LConn3 -- Bus 8/LConn1
  Bus 5/RConn3 -- C5_6/RConn1 -- Distributed Parameters Line3/RConn1
  Bus 5/RConn2 -- B5_6/RConn1 -- Distributed Parameters Line3/RConn2
  Bus 5/RConn1 -- Distributed Parameters Line3/RConn3 -- A5_6/RConn1
  "GT 1 "/RConn3 -- Bus 39/RConn3 -- Load 39/LConn3 -- C39/RConn1
  "GT 1 "/RConn2 -- Load 39/LConn2 -- Bus 39/RConn2 -- B39/RConn1
  Bus 39/RConn1 -- "GT 1 "/RConn1 -- A39/RConn1 -- Load 39/LConn1
  Load Flow Bus8/LConn1 -- Distributed Parameters Line9/RConn1 -- Bus 39/LConn1
  Distributed Parameters Line9/RConn2 -- Bus 39/LConn2
  Distributed Parameters Line9/RConn3 -- Bus 39/LConn3
  Bus 9/LConn1 -- Distributed Parameters Line1/RConn3
  Distributed Parameters Line1/RConn2 -- Bus 9/LConn2
  Bus 9/LConn3 -- Distributed Parameters Line1/RConn1
  Distributed Parameters Line2/RConn1 -- Bus 5/LConn1
  Distributed Parameters Line2/RConn2 -- Bus 5/LConn2
  Load Flow Bus2/LConn1 -- Distributed Parameters Line2/RConn3 -- Bus 5/LConn3
  Load Flow Bus1/LConn1 -- Distributed Parameters Line3/LConn3 -- Bus 4/LConn1
  Bus 4/LConn2 -- Distributed Parameters Line3/LConn2
  Bus 4/LConn3 -- Distributed Parameters Line3/LConn1
  B4_3/RConn1 -- B4_14/RConn1 -- Load 4/LConn2 -- Bus 4/RConn2
  A4_3/RConn1 -- A4_14/RConn1 -- Load 4/LConn1 -- Bus 4/RConn1
  C4_3/RConn1 -- C4_14/RConn1 -- Load 4/LConn3 -- Bus 4/RConn3
